simulink library "QuaternionLib"  (R2014b)
settings: Solver=ode45  StartTime=0.0  StopTime=10.0  RelTol=1e-3
libraries: QuaternionLib x10
settings Model: Creator=Ewing  LastModifiedBy=5909

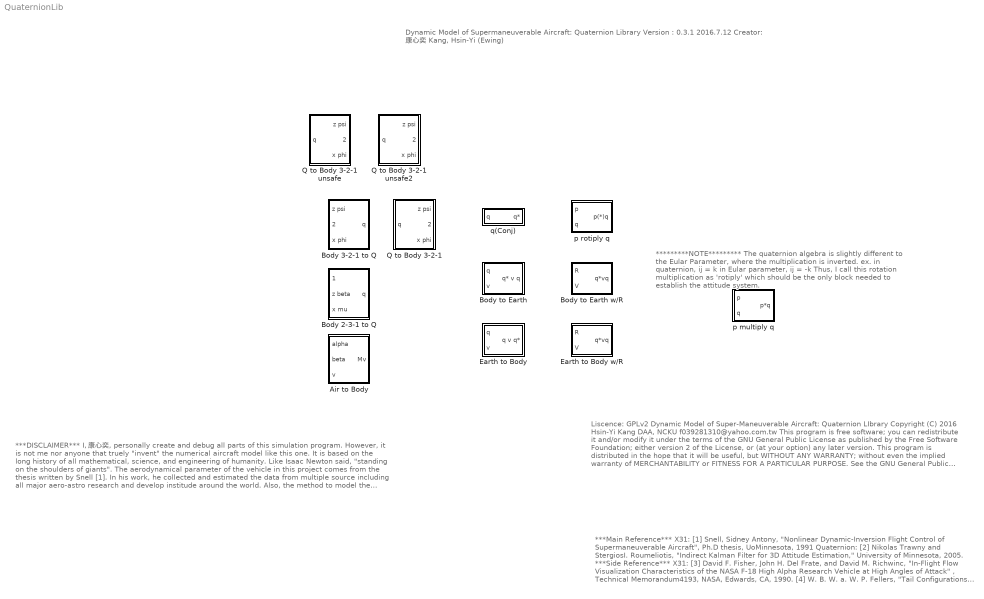
== system QuaternionLib ==
  note: *********NOTE*********
      | The quaternion algebra is slightly different to
      | the Eular Parameter, where the multiplication is inverted.
      | 	ex. 	in quaternion, ij = k
      | 		in Eular parameter, ij = -k
      | Thus, I call this rotation multiplication as 'rotiply' which should
      |  be the only block needed to establish the attitude system.
  note: Liscence: GPLv2
      | Dynamic Model of Super-Maneuverable Aircraft: Quaternion LIbrary
      | Copyright (C) 2016 Hsin-Yi Kang
      | DAA, NCKU
      | f039281310@yahoo.com.tw
      | This program is free software; you can redistribute it and/or modify it under the terms of the GNU General Public License as published by the Free Software Foundation; either version 2 of the License, or (at your option) any later version. This program is distributed in the hope that it will be useful, but WITHOUT ANY WARRANTY; without even the implied warranty of MERCHANTABILITY or FITNESS FOR A PARTICULAR PURPOSE. See the GNU General Public License for more details. You should have received a copy of the GNU General Public License along with this program; if not, write to the Free Software Foundation, Inc., 51 Franklin Street, Fifth Floor, Boston, MA 02110-1301, USA.
  note: ***DISCLAIMER***
      | I, 康心奕, personally create and debug all parts of this simulation program. However, it is not me nor anyone that truely "invent" the numerical aircraft model like this one. It is based on the long history of all mathematical, science, and engineering of humanity. Like Isaac Newton said, "standing on the shoulders of giants".
      | The aerodynamical parameter of the vehicle in this project comes from the thesis written by Snell [1]. In his work, he collected and estimated the data from multiple source including all major aero-astro research and develop institude around the world. Also, the method to model the dynamics of the vehicle and the controller implemented including the NDI and Gain Scheduling also came from his thesis.
      | The quaternion kinematics mainly reference to the toturial paper done by Trawny [2], where he collected and organized all fundamental properties and mathematical operation of such system.
      | This model is released to improve our ability to understand and develop control methodology of aerial vehicle system similar to this one. It is released free of charge now and always will be so in the hope of sharing the knowledge as much as possible and making this world a better place.
      | However, despite my greatest effort to ensure the correctness of the code, it is not garantee to be free of bug or other issue. You are free to use and modify the program to meet your need but I'm not responsible for any potential risk or damaged of any kind.
      |
      | Long live and prosper
  note: ***Main Reference***
      | X31:
      | [1] Snell, Sidney Antony, "Nonlinear Dynamic-Inversion Flight Control of Supermaneuverable Aircraft", Ph.D thesis, UoMinnesota, 1991
      | Quaternion:
      | [2] Nikolas Trawny and StergiosI. Roumeliotis, "Indirect Kalman Filter for 3D Attitude Estimation," University of Minnesota, 2005.
      |
      | ***Side Reference***
      | X31:
      | [3] David F. Fisher, John H. Del Frate, and David M. Richwinc, "In-Flight Flow Visualization Characteristics of the NASA F-18 High Alpha Research Vehicle at High Angles of Attack"
      | , Technical Memorandum4193, NASA, Edwards, CA, 1990.
      | [4] W. B. W. a. W. P. Fellers, "Tail Configurations for Highly Maneuverable Aircraft," AGARD, 1981.
      |
      | Quaternion:
      | [5] Nikolas Trawnyand StergiosI. Roumeliotis, "Indirect Kalman Filter for 3D Attitude Estimation," University of Minnesota, 2005.
      | [6] W. G. Breckenridge, "Quaternions -Proposed Standard Conventions," JPL, Tech. Rep. INTEROFFICE MEMORANDUM 343-79-1199, 1999.
      | [7] D. M. Henderson, "EularAngles, Quaternions, and Transformation Matrices," Mission Planning and Analysis Division, NASA, July 1977.
  note: Dynamic Model of Supermaneuverable Aircraft: Quaternion Library
      | Version : 0.3.1
      | 2016.7.12
      | Creator: 康心奕 Kang, Hsin-Yi (Ewing)
  Air to Body : Subsystem
      mask help: Earth to body by rotational matrix Mv
  Body 2-3-1 to Q : Subsystem
      mask help: Given a Body 3-2-1 rotation, and it'll find its corresponding quaternion
  Body 3-2-1 to Q : Subsystem
      mask help: Given a Body 3-2-1 rotation, and it'll find its corresponding quaternion
  Body to Earth : Subsystem
      mask help: Body to Earth is Q*VQ
  Body to Earth w/R : Subsystem
      mask help: Express a veter define in body frame in earth frame
  Earth to Body : Subsystem
      mask help: Earth to body is QVQ*
  Earth to Body w/R : Subsystem
      mask help: Express a veter define in earth frame in body frame
  Q to Body 3-2-1 : Subsystem
      mask help: Given a Body 3-2-1 rotation, and it'll find its corresponding quaternion
  Q to Body 3-2-1 unsafe : Subsystem
      mask help: Given a Body 3-2-1 rotation, and it'll find its corresponding quaternion
  Q to Body 3-2-1 unsafe2 : Subsystem
      mask help: Given a Body 3-2-1 rotation, and it'll find its corresponding quaternion
  p multiply q : Subsystem
      mask help: The true multiply of a quaternion.
  p rotiply q : Subsystem
      mask help:
      | Quaternion p mulpiply q
      | This means a orientation q is rotate by p consecutively
      | Note this is not as same as a normal quaternion multiply method in order to improve readability of the quaternion.
  q(Conj) : Subsystem
      mask help: Quaternion conjugate

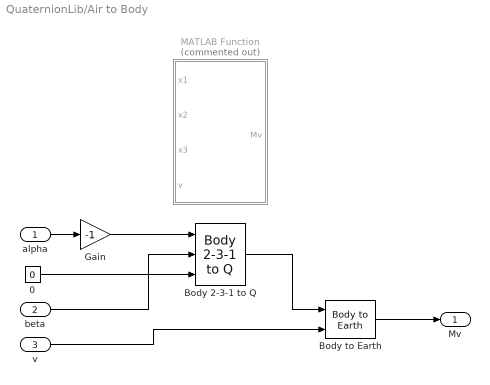
== system QuaternionLib/Air to Body ==
  alpha : Inport
  beta : Inport  Port=2
  v : Inport  Port=3
  0 : Constant  Value=0
  Body 2-3-1 to Q : QuaternionLib/Body 2-3-1 to Q
  Body to Earth : QuaternionLib/Body to Earth
  Gain : Gain  Gain=-1
  MATLAB Function : MATLAB Function  Commented=on  TreatAsAtomicUnit=on
  Mv : Outport
  wires:
  Body to Earth/1 -> Mv/1
  alpha/1 -> Gain/1
  beta/1 -> Body 2-3-1 to Q/2
  0/1 -> Body 2-3-1 to Q/3
  v/1 -> Body to Earth/2
  Gain/1 -> Body 2-3-1 to Q/1
  Body 2-3-1 to Q/1 -> Body to Earth/1

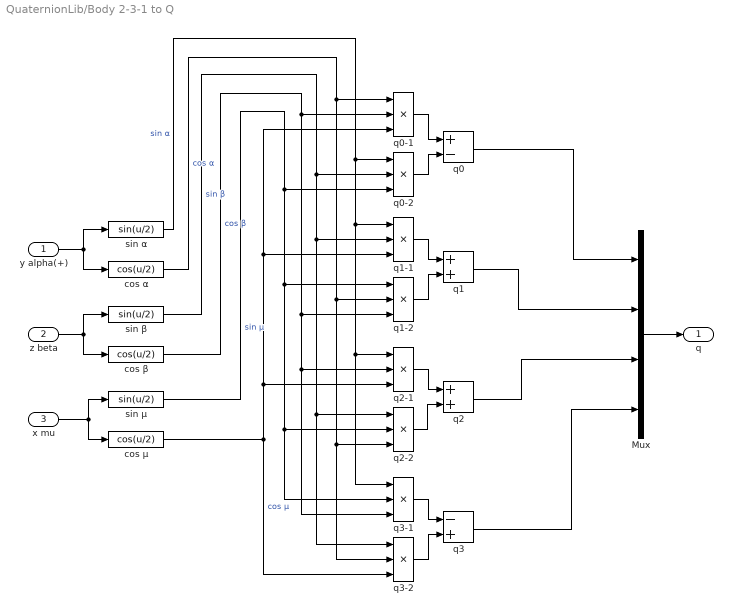
== system QuaternionLib/Body 2-3-1 to Q ==
  y alpha(+) : Inport
  z beta : Inport  Port=2
  x mu : Inport  Port=3
  Mux : Mux
  cos α : Fcn  Expr=cos(u/2)
  cos β : Fcn  Expr=cos(u/2)
  cos μ : Fcn  Expr=cos(u/2)
  q0 : Sum  Inputs=+-
  q0-1 : Product  Inputs=3
  q0-2 : Product  Inputs=3
  q1 : Sum
  q1-1 : Product  Inputs=3
  q1-2 : Product  Inputs=3
  q2 : Sum
  q2-1 : Product  Inputs=3
  q2-2 : Product  Inputs=3
  q3 : Sum  Inputs=-+
  q3-1 : Product  Inputs=3
  q3-2 : Product  Inputs=3
  sin α : Fcn  Expr=sin(u/2)
  sin β : Fcn  Expr=sin(u/2)
  sin μ : Fcn  Expr=sin(u/2)
  q : Outport
  wires:
  y alpha(+)/1 -> sin α/1, cos α/1
  z beta/1 -> sin β/1, cos β/1
  x mu/1 -> cos μ/1, sin μ/1
  cos α/1 -> q1-2/2, q3-2/2, q2-2/3, q0-1/1  "cos α"
  cos β/1 -> q1-2/3, q3-1/3, q2-1/2, q0-1/2  "cos β"
  cos μ/1 -> q2-1/3, q1-1/3, q0-1/3, q3-2/3  "cos μ"
  sin α/1 -> q1-1/1, q3-1/1, q2-1/1, q0-2/1  "sin α"
  sin β/1 -> q1-1/2, q3-2/1, q2-2/1, q0-2/2  "sin β"
  sin μ/1 -> q1-2/1, q2-2/2, q3-1/2, q0-2/3  "sin μ"
  q0-1/1 -> q0/1
  q0-2/1 -> q0/2
  q1-1/1 -> q1/1
  q1-2/1 -> q1/2
  q2-1/1 -> q2/1
  q2-2/1 -> q2/2
  q3-1/1 -> q3/1
  q3-2/1 -> q3/2
  q0/1 -> Mux/1
  q1/1 -> Mux/2
  q2/1 -> Mux/3
  q3/1 -> Mux/4
  Mux/1 -> q/1

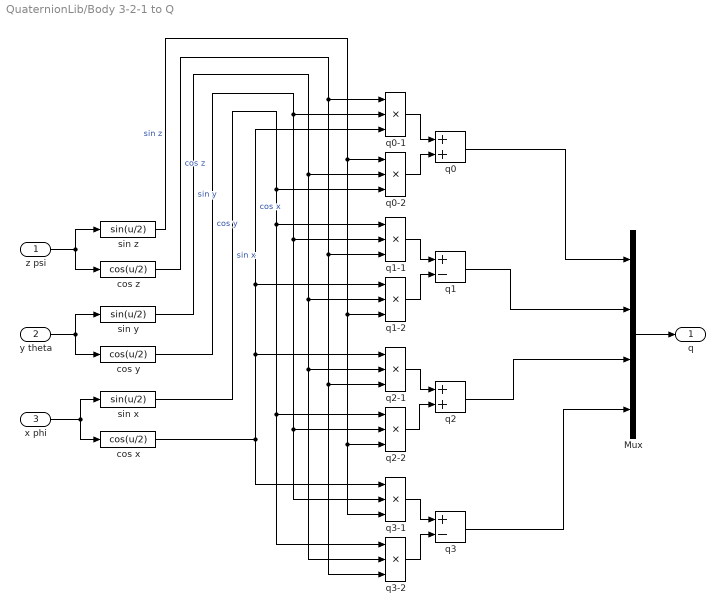
== system QuaternionLib/Body 3-2-1 to Q ==
  z psi : Inport
  y theta : Inport  Port=2
  x phi : Inport  Port=3
  Mux : Mux
  cos x : Fcn  Expr=cos(u/2)
  cos y : Fcn  Expr=cos(u/2)
  cos z : Fcn  Expr=cos(u/2)
  q0 : Sum
  q0-1 : Product  Inputs=3
  q0-2 : Product  Inputs=3
  q1 : Sum  Inputs=+-
  q1-1 : Product  Inputs=3
  q1-2 : Product  Inputs=3
  q2 : Sum
  q2-1 : Product  Inputs=3
  q2-2 : Product  Inputs=3
  q3 : Sum  Inputs=+-
  q3-1 : Product  Inputs=3
  q3-2 : Product  Inputs=3
  sin x : Fcn  Expr=sin(u/2)
  sin y : Fcn  Expr=sin(u/2)
  sin z : Fcn  Expr=sin(u/2)
  q : Outport
  wires:
  z psi/1 -> sin z/1, cos z/1
  y theta/1 -> sin y/1, cos y/1
  x phi/1 -> cos x/1, sin x/1
  cos z/1 -> q3-2/3, q2-1/3, q1-1/3, q0-1/1  "cos z"
  cos y/1 -> q3-1/2, q2-2/2, q1-1/2, q0-1/2  "cos y"
  cos x/1 -> q3-1/1, q0-1/3, q1-2/1, q2-1/1  "cos x"
  sin z/1 -> q3-1/3, q2-2/3, q1-2/3, q0-2/1  "sin z"
  sin y/1 -> q3-2/2, q2-1/2, q1-2/2, q0-2/2  "sin y"
  sin x/1 -> q3-2/1, q2-2/1, q1-1/1, q0-2/3  "sin x"
  q0-1/1 -> q0/1
  q0-2/1 -> q0/2
  q1-1/1 -> q1/1
  q1-2/1 -> q1/2
  q2-1/1 -> q2/1
  q2-2/1 -> q2/2
  q3-1/1 -> q3/1
  q3-2/1 -> q3/2
  q0/1 -> Mux/1
  q1/1 -> Mux/2
  q2/1 -> Mux/3
  q3/1 -> Mux/4
  Mux/1 -> q/1

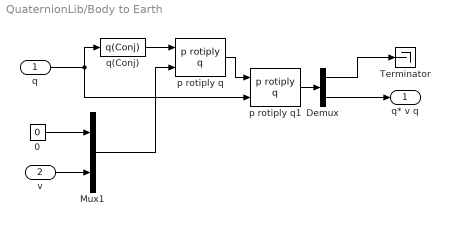
== system QuaternionLib/Body to Earth ==
  q : Inport
  v : Inport  Port=2
  0 : Constant  Value=0
  Demux : Demux  Outputs=[1 3]
  Mux1 : Mux  Inputs=2
  Terminator : Terminator
  p rotiply q : QuaternionLib/p rotiply q
  p rotiply q1 : QuaternionLib/p rotiply q
  q(Conj) : QuaternionLib/q(Conj)
  q* v q : Outport
  wires:
  v/1 -> Mux1/2
  0/1 -> Mux1/1
  q/1 -> p rotiply q1/2, q(Conj)/1
  Mux1/1 -> p rotiply q/2
  p rotiply q1/1 -> Demux/1
  q(Conj)/1 -> p rotiply q/1
  Demux/1 -> Terminator/1
  Demux/2 -> q* v q/1
  p rotiply q/1 -> p rotiply q1/1

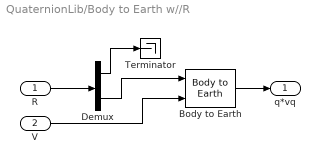
== system QuaternionLib/Body to Earth w//R ==
  R : Inport
  V : Inport  Port=2
  Body to Earth : QuaternionLib/Body to Earth
  Demux : Demux  Outputs=[3 4]
  Terminator : Terminator
  q*vq : Outport
  wires:
  Body to Earth/1 -> q*vq/1
  R/1 -> Demux/1
  V/1 -> Body to Earth/2
  Demux/2 -> Body to Earth/1
  Demux/1 -> Terminator/1

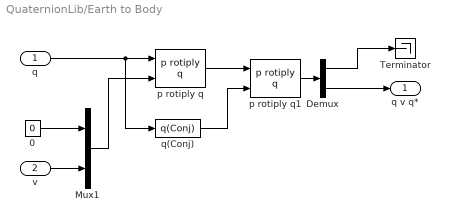
== system QuaternionLib/Earth to Body ==
  q : Inport
  v : Inport  Port=2
  0 : Constant  Value=0
  Demux : Demux  Outputs=[1 3]
  Mux1 : Mux  Inputs=2
  Terminator : Terminator
  p rotiply q : QuaternionLib/p rotiply q
  p rotiply q1 : QuaternionLib/p rotiply q
  q(Conj) : QuaternionLib/q(Conj)
  q v q* : Outport
  wires:
  v/1 -> Mux1/2
  0/1 -> Mux1/1
  q/1 -> p rotiply q/1, q(Conj)/1
  Mux1/1 -> p rotiply q/2
  p rotiply q/1 -> p rotiply q1/1
  q(Conj)/1 -> p rotiply q1/2
  p rotiply q1/1 -> Demux/1
  Demux/1 -> Terminator/1
  Demux/2 -> q v q*/1

== system QuaternionLib/Earth to Body w//R ==
  R : Inport
  V : Inport  Port=2
  Demux : Demux  Outputs=[3 4]
  Earth to Body : QuaternionLib/Earth to Body
  Terminator : Terminator
  q*vq : Outport
  wires:
  Earth to Body/1 -> q*vq/1
  R/1 -> Demux/1
  V/1 -> Earth to Body/2
  Demux/2 -> Earth to Body/1
  Demux/1 -> Terminator/1

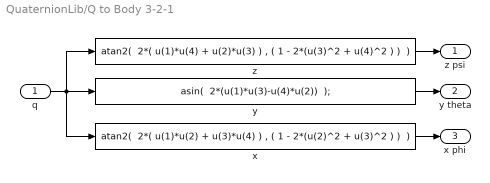
== system QuaternionLib/Q to Body 3-2-1 ==
  q : Inport
  x : Fcn  Expr="atan2(  2*( u(1)*u(2) + u(3)*u(4) ) , ( 1 - 2*(u(2)^2 + u(3)^2 ) )  )"
  y : Fcn  Expr="asin(  2*(u(1)*u(3)-u(4)*u(2))  );"
  z : Fcn  Expr="atan2(  2*( u(1)*u(4) + u(2)*u(3) ) , ( 1 - 2*(u(3)^2 + u(4)^2 ) )  )"
  z psi : Outport
  y theta : Outport  Port=2
  x phi : Outport  Port=3
  wires:
  q/1 -> z/1, x/1, y/1
  z/1 -> z psi/1
  y/1 -> y theta/1
  x/1 -> x phi/1

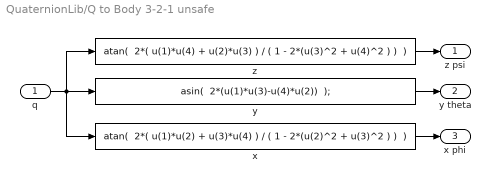
== system QuaternionLib/Q to Body 3-2-1 unsafe ==
  q : Inport
  x : Fcn  Expr="atan(  2*( u(1)*u(2) + u(3)*u(4) ) / ( 1 - 2*(u(2)^2 + u(3)^2 ) )  )"
  y : Fcn  Expr="asin(  2*(u(1)*u(3)-u(4)*u(2))  );"
  z : Fcn  Expr="atan(  2*( u(1)*u(4) + u(2)*u(3) ) / ( 1 - 2*(u(3)^2 + u(4)^2 ) )  )"
  z psi : Outport
  y theta : Outport  Port=2
  x phi : Outport  Port=3
  wires:
  q/1 -> z/1, x/1, y/1
  z/1 -> z psi/1
  y/1 -> y theta/1
  x/1 -> x phi/1

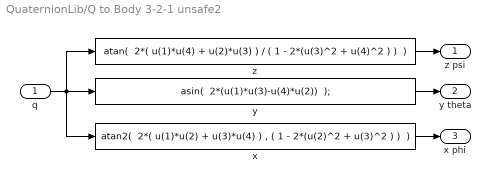
== system QuaternionLib/Q to Body 3-2-1 unsafe2 ==
  q : Inport
  x : Fcn  Expr="atan2(  2*( u(1)*u(2) + u(3)*u(4) ) , ( 1 - 2*(u(2)^2 + u(3)^2 ) )  )"
  y : Fcn  Expr="asin(  2*(u(1)*u(3)-u(4)*u(2))  );"
  z : Fcn  Expr="atan(  2*( u(1)*u(4) + u(2)*u(3) ) / ( 1 - 2*(u(3)^2 + u(4)^2 ) )  )"
  z psi : Outport
  y theta : Outport  Port=2
  x phi : Outport  Port=3
  wires:
  q/1 -> z/1, x/1, y/1
  z/1 -> z psi/1
  y/1 -> y theta/1
  x/1 -> x phi/1

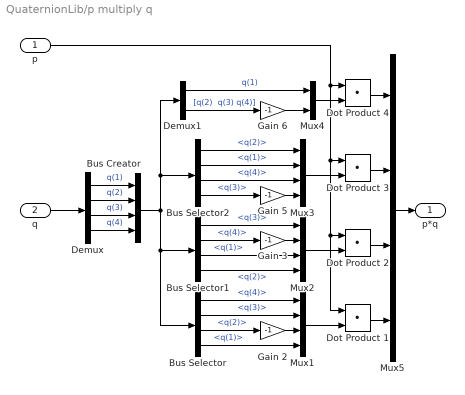
== system QuaternionLib/p multiply q ==
  p : Inport  PortDimensions=4
  q : Inport  Port=2  PortDimensions=4
  Bus Creator : BusCreator
  Bus Selector : BusSelector  OutputSignals=q(4),q(3),q(2),q(1)
  Bus Selector1 : BusSelector  OutputSignals=q(3),q(4),q(1),q(2)
  Bus Selector2 : BusSelector  OutputSignals=q(2),q(1),q(4),q(3)
  Demux : Demux
  Demux1 : Demux  Outputs=[1 3]
  Dot Product {1..4} (4 alike) : DotProduct  InputSameDT=on  OutDataTypeStr=Inherit: Inherit via internal rule
  Gain {2..3,5..6} (4 alike) : Gain  Gain=-1  SaturateOnIntegerOverflow=on  OutDataTypeStr=Inherit: Same as input  ParamDataTypeStr=Inherit: Same as input
  Mux{1..3,5} (4 alike) : Mux
  Mux4 : Mux  Inputs=2
  p*q : Outport
  wires:
  Dot Product 1/1 -> Mux5/4
  Gain 3/1 -> Mux2/2
  Dot Product 2/1 -> Mux5/3
  Gain 5/1 -> Mux3/4
  Dot Product 3/1 -> Mux5/2
  Gain 6/1 -> Mux4/2
  p/1 -> Dot Product 1/1, Dot Product 2/1, Dot Product 3/1, Dot Product 4/1
  Bus Creator/1 -> Bus Selector1/1, Bus Selector/1, Demux1/1, Bus Selector2/1
  Dot Product 4/1 -> Mux5/1
  Demux/4 -> Bus Creator/4  "q(4)"
  Demux/3 -> Bus Creator/3  "q(3)"
  Demux/2 -> Bus Creator/2  "q(2)"
  Demux/1 -> Bus Creator/1  "q(1)"
  Mux5/1 -> p*q/1
  Mux3/1 -> Dot Product 3/2
  Mux2/1 -> Dot Product 2/2
  Mux1/1 -> Dot Product 1/2
  Bus Selector2/3 -> Mux3/3  "<q(4)>"
  Bus Selector1/2 -> Gain 3/1  "<q(4)>"
  Bus Selector/1 -> Mux1/1  "<q(4)>"
  Bus Selector/2 -> Mux1/2  "<q(3)>"
  Bus Selector/3 -> Gain 2/1  "<q(2)>"
  Gain 2/1 -> Mux1/3
  Bus Selector/4 -> Mux1/4  "<q(1)>"
  Bus Selector1/1 -> Mux2/1  "<q(3)>"
  Bus Selector1/3 -> Mux2/3  "<q(1)>"
  Bus Selector1/4 -> Mux2/4  "<q(2)>"
  Bus Selector2/2 -> Mux3/2  "<q(1)>"
  Bus Selector2/1 -> Mux3/1  "<q(2)>"
  Bus Selector2/4 -> Gain 5/1  "<q(3)>"
  Mux4/1 -> Dot Product 4/2
  Demux1/1 -> Mux4/1  "q(1)"
  Demux1/2 -> Gain 6/1  "[q(2)  q(3) q(4)]"
  q/1 -> Demux/1

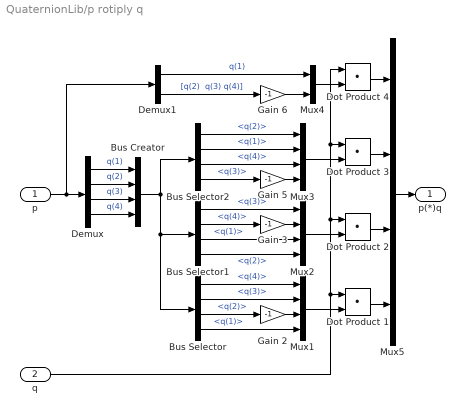
== system QuaternionLib/p rotiply q ==
  p : Inport  PortDimensions=4
  q : Inport  Port=2  PortDimensions=4
  Bus Creator : BusCreator
  Bus Selector : BusSelector  OutputSignals=q(4),q(3),q(2),q(1)
  Bus Selector1 : BusSelector  OutputSignals=q(3),q(4),q(1),q(2)
  Bus Selector2 : BusSelector  OutputSignals=q(2),q(1),q(4),q(3)
  Demux : Demux
  Demux1 : Demux  Outputs=[1 3]
  Dot Product {1..4} (4 alike) : DotProduct  InputSameDT=on  OutDataTypeStr=Inherit: Inherit via internal rule
  Gain {2..3,5..6} (4 alike) : Gain  Gain=-1  SaturateOnIntegerOverflow=on  OutDataTypeStr=Inherit: Same as input  ParamDataTypeStr=Inherit: Same as input
  Mux{1..3,5} (4 alike) : Mux
  Mux4 : Mux  Inputs=2
  p(*)q : Outport
  wires:
  Dot Product 1/1 -> Mux5/4
  Gain 3/1 -> Mux2/2
  Dot Product 2/1 -> Mux5/3
  Gain 5/1 -> Mux3/4
  Dot Product 3/1 -> Mux5/2
  Gain 6/1 -> Mux4/2
  q/1 -> Dot Product 4/1, Dot Product 3/1, Dot Product 2/1, Dot Product 1/1
  Bus Creator/1 -> Bus Selector1/1, Bus Selector/1, Bus Selector2/1
  Dot Product 4/1 -> Mux5/1
  Demux/4 -> Bus Creator/4  "q(4)"
  Demux/3 -> Bus Creator/3  "q(3)"
  Demux/2 -> Bus Creator/2  "q(2)"
  Demux/1 -> Bus Creator/1  "q(1)"
  Mux5/1 -> p(*)q/1
  Mux3/1 -> Dot Product 3/2
  Mux2/1 -> Dot Product 2/2
  Mux1/1 -> Dot Product 1/2
  Bus Selector2/3 -> Mux3/3  "<q(4)>"
  Bus Selector1/2 -> Gain 3/1  "<q(4)>"
  Bus Selector/1 -> Mux1/1  "<q(4)>"
  Bus Selector/2 -> Mux1/2  "<q(3)>"
  Bus Selector/3 -> Gain 2/1  "<q(2)>"
  Gain 2/1 -> Mux1/3
  Bus Selector/4 -> Mux1/4  "<q(1)>"
  Bus Selector1/1 -> Mux2/1  "<q(3)>"
  Bus Selector1/3 -> Mux2/3  "<q(1)>"
  Bus Selector1/4 -> Mux2/4  "<q(2)>"
  Bus Selector2/2 -> Mux3/2  "<q(1)>"
  Bus Selector2/1 -> Mux3/1  "<q(2)>"
  Bus Selector2/4 -> Gain 5/1  "<q(3)>"
  Mux4/1 -> Dot Product 4/2
  Demux1/1 -> Mux4/1  "q(1)"
  Demux1/2 -> Gain 6/1  "[q(2)  q(3) q(4)]"
  p/1 -> Demux1/1, Demux/1

== system QuaternionLib/q(Conj) ==
  q : Inport  PortDimensions=4
  Demux : Demux  Outputs=[1 3]
  Gain : Gain  Gain=-1  SaturateOnIntegerOverflow=on  OutDataTypeStr=Inherit: Same as input  ParamDataTypeStr=Inherit: Same as input
  Mux : Mux  Inputs=2
  q* : Outport
  wires:
  Gain/1 -> Mux/2
  Mux/1 -> q*/1
  Demux/2 -> Gain/1  "[q(2)  q(3) q(4)]"
  Demux/1 -> Mux/1  "q(1)"
  q/1 -> Demux/1

== matlab function QuaternionLib/Air to Body/MATLAB Function ==
  data: x1 input; Mv output; x2 input; x3 input; v input
function Mv = body321_tf(x1, x2, x3, v)
c1 = cos(x3);
s1 = sin(x3);
c2 = cos(x2);
s2 = sin(x2);
c3 = cos(x1);
s3 = sin(x1);
M = [   c1*c2 , c1*s2*s3 - c3*s1 , c1*s2*c3 + s3*s1 ;...
        s1*c2 , s1*s2*s3 + c3*c1 , s1*s2*c3 - s3*c1 ;...
        -s2   ,            c2*s3 ,            c2*c3     ];
Mv = (M * v) ;
end
